simulink model "Aerodynamicsyuan"  (R2017b)
settings: Solver=VariableStepAuto  StartTime=0.0  StopTime=10.0  RelTol=1e-3
values from neighbouring files (symbols this model uses):
  CDAlpha = 0.10031    [aerodata.m]
  CDBeta = 8.0356e-06    [aerodata.m]
  CDDa = 1.3547e-05    [aerodata.m]
  CDDe = 0.020779    [aerodata.m]
  CDDf = 0.031301    [aerodata.m]
  CDDr = 1.437e-05    [aerodata.m]
  CLAlpha = 6.0094    [aerodata.m]
  ClAlpha = -4.2668e-14    [aerodata.m]
  CLBeta = -1.0202e-06    [aerodata.m]
  ClBeta = 0.055654    [aerodata.m]
  CLDa = 2.6815e-06    [aerodata.m]
  ClDa = 0.29533    [aerodata.m]
  CLDe = 0.8867    [aerodata.m]
  CLDf = 2.0336    [aerodata.m]
  CLDr = -3.5351e-06    [aerodata.m]
  ClDr = 0.29533    [aerodata.m]
  CmAlpha = -4.0835    [aerodata.m]
  CmBeta = 5.2248e-06    [aerodata.m]
  CmDa = 1.0717e-06    [aerodata.m]
  CmDe = -2.7271    [aerodata.m]
  CmDf = -0.35441    [aerodata.m]
  CmDr = 1.0717e-06    [aerodata.m]
  CnAlpha = 4.5786e-14    [aerodata.m]
  CnBeta = -0.071639    [aerodata.m]
  CnDa = 0.0089298    [aerodata.m]
  CnDr = -0.10037    [aerodata.m]
  CYAlpha = 8.85452e-14    [aerodata.m]
  CYBeta = -0.25081    [aerodata.m]
  CYDa = 0.0029468    [aerodata.m]
  CYDe = 9.0523e-14    [aerodata.m]
  CYDf = 9.8247e-14    [aerodata.m]
  CYDr = -0.33334    [aerodata.m]
libraries: aerolibatmos2 x1
settings Model: Creator=zht  LastModifiedBy=p'c

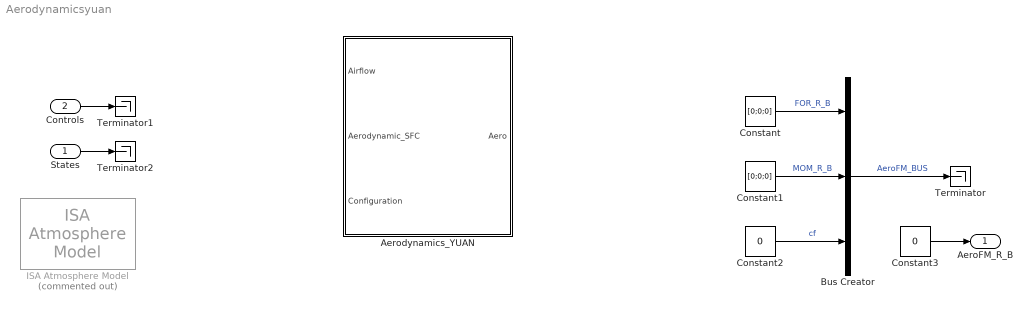
== system Aerodynamicsyuan ==
  States : Inport
  Controls : Inport  Port=2
  Aerodynamics_YUAN : Subsystem
  Bus Creator : BusCreator  Inputs=3
  Constant : Constant  Value=[0;0;0]
  Constant1 : Constant  Value=[0;0;0]
  Constant2 : Constant  Value=0
  Constant3 : Constant  Value=0
  ISA Atmosphere Model : aerolibatmos2/ISA Atmosphere Model  Commented=on  custom=off  g=9.80665  gamma=1.4  R=287.0531  L=0.0065  h_trop=11000  h_strat=20000  rho0=1.225  P0=101325  T0=288.15  h0=0
      settings: SourceProductName=Aerospace Blockset
  Terminator : Terminator
  Terminator1 : Terminator
  Terminator2 : Terminator
  AeroFM_R_B : Outport
  wires:
  Bus Creator/1 -> Terminator/1  "AeroFM_BUS"
  Constant2/1 -> Bus Creator/3  "cf"
  Constant1/1 -> Bus Creator/2  "MOM_R_B"
  Constant/1 -> Bus Creator/1  "FOR_R_B"
  Constant3/1 -> AeroFM_R_B/1
  Controls/1 -> Terminator1/1
  States/1 -> Terminator2/1

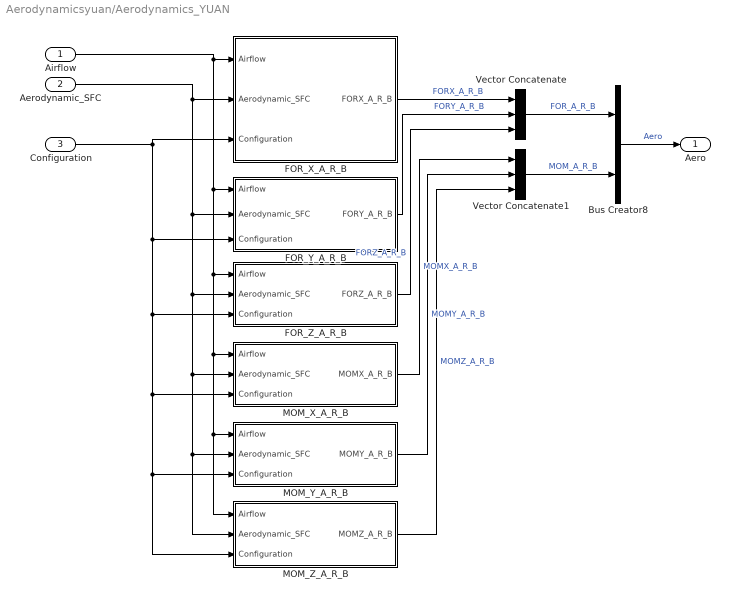
== system Aerodynamicsyuan/Aerodynamics_YUAN ==
  Airflow : Inport  OutDataTypeStr=Bus: Airflow_BUS  BusOutputAsStruct=on
  Aerodynamic_SFC : Inport  Port=2  OutDataTypeStr=Bus: DEF_Aero_SFC_Deflections_BUS  BusOutputAsStruct=on
  Configuration : Inport  Port=3  OutDataTypeStr=Bus: Configuration_BUS  BusOutputAsStruct=on
  Bus Creator8 : BusCreator  Inputs='FOR_A_R_B','MOM_A_R_B'  OutDataTypeStr=Bus: Aero_BUS  NonVirtualBus=on
  FOR_X_A_R_B : Subsystem
  FOR_Y_A_R_B : Subsystem
  FOR_Z_A_R_B : Subsystem
  MOM_X_A_R_B : Subsystem
  MOM_Y_A_R_B : Subsystem
  MOM_Z_A_R_B : Subsystem
  Vector Concatenate : Concatenate  NumInputs=3  Mode=Multidimensional array
  Vector Concatenate1 : Concatenate  NumInputs=3  Mode=Multidimensional array
  Aero : Outport  OutDataTypeStr=Bus: Aero_BUS  BusOutputAsStruct=on
  wires:
  FOR_Y_A_R_B/1(FORY_A_R_B) -> Vector Concatenate/2  "FORY_A_R_B"
  MOM_Z_A_R_B/1(MOMZ_A_R_B) -> Vector Concatenate1/3  "MOMZ_A_R_B"
  MOM_Y_A_R_B/1(MOMY_A_R_B) -> Vector Concatenate1/2  "MOMY_A_R_B"
  Aerodynamic_SFC/1 -> FOR_X_A_R_B/2(Aerodynamic_SFC), FOR_Y_A_R_B/2(Aerodynamic_SFC), FOR_Z_A_R_B/2(Aerodynamic_SFC), MOM_X_A_R_B/2(Aerodynamic_SFC), MOM_Y_A_R_B/2(Aerodynamic_SFC), MOM_Z_A_R_B/2(Aerodynamic_SFC)
  FOR_Z_A_R_B/1(FORZ_A_R_B) -> Vector Concatenate/3  "FORZ_A_R_B"
  Vector Concatenate1/1 -> Bus Creator8/2  "MOM_A_R_B"
  Vector Concatenate/1 -> Bus Creator8/1  "FOR_A_R_B"
  Bus Creator8/1 -> Aero/1  "Aero"
  MOM_X_A_R_B/1(MOMX_A_R_B) -> Vector Concatenate1/1  "MOMX_A_R_B"
  FOR_X_A_R_B/1(FORX_A_R_B) -> Vector Concatenate/1  "FORX_A_R_B"
  Airflow/1 -> FOR_X_A_R_B/1(Airflow), FOR_Y_A_R_B/1(Airflow), FOR_Z_A_R_B/1(Airflow), MOM_X_A_R_B/1(Airflow), MOM_Y_A_R_B/1(Airflow), MOM_Z_A_R_B/1(Airflow)
  Configuration/1 -> FOR_X_A_R_B/3(Configuration), FOR_Y_A_R_B/3(Configuration), FOR_Z_A_R_B/3(Configuration), MOM_X_A_R_B/3(Configuration), MOM_Y_A_R_B/3(Configuration), MOM_Z_A_R_B/3(Configuration)

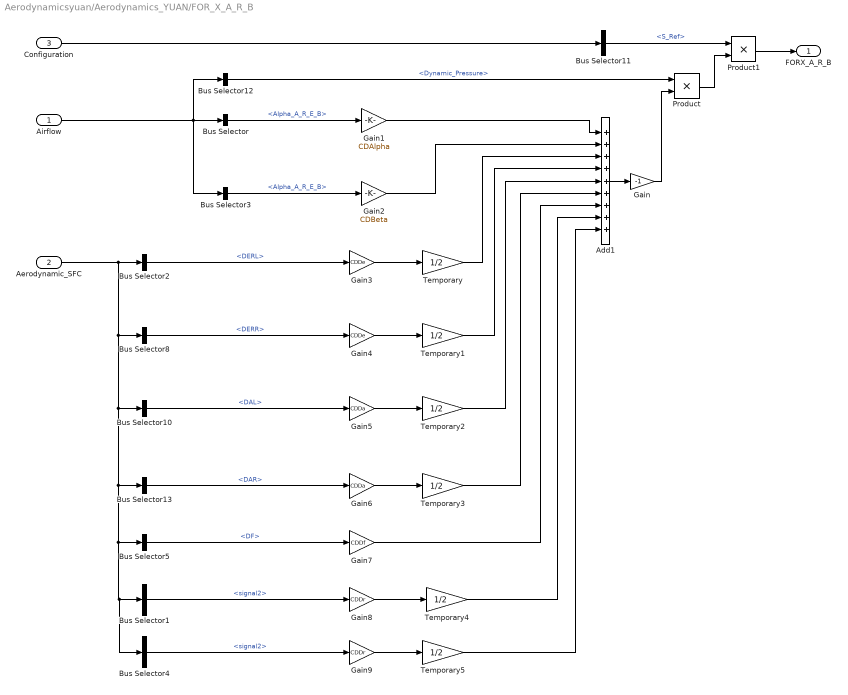
== system Aerodynamicsyuan/Aerodynamics_YUAN/FOR_X_A_R_B ==
  Airflow : Inport  OutDataTypeStr=Bus: Airflow_BUS  BusOutputAsStruct=on
  Aerodynamic_SFC : Inport  Port=2  OutDataTypeStr=Bus: DEF_Aero_SFC_Deflections_BUS  BusOutputAsStruct=on
  Configuration : Inport  Port=3  OutDataTypeStr=Bus: Configuration_BUS  BusOutputAsStruct=on
  Add1 : Sum  Inputs=+++++++++
  Bus Selector : BusSelector  OutputSignals=Alpha_A_R_E_B
  Bus Selector1 : BusSelector  OutputSignals=signal2
  Bus Selector10 : BusSelector  OutputSignals=DAL
  Bus Selector11 : BusSelector  OutputSignals=S_Ref
  Bus Selector12 : BusSelector  OutputSignals=Dynamic_Pressure
  Bus Selector13 : BusSelector  OutputSignals=DAR
  Bus Selector2 : BusSelector  OutputSignals=DERL
  Bus Selector3 : BusSelector  OutputSignals=Alpha_A_R_E_B
  Bus Selector4 : BusSelector  OutputSignals=signal2
  Bus Selector5 : BusSelector  OutputSignals=DF
  Bus Selector8 : BusSelector  OutputSignals=DERR
  Gain : Gain  Gain=-1
  Gain1 : Gain  Gain=CDAlpha
  Gain2 : Gain  Gain=CDBeta
  Gain3 : Gain  Gain=CDDe
  Gain4 : Gain  Gain=CDDe
  Gain5 : Gain  Gain=CDDa
  Gain6 : Gain  Gain=CDDa
  Gain7 : Gain  Gain=CDDf
  Gain8 : Gain  Gain=CDDr
  Gain9 : Gain  Gain=CDDr
  Product : Product
  Product1 : Product
  Temporary{,1..5} (6 alike) : Gain  Gain=1/2
  FORX_A_R_B : Outport  Unit=N  PortDimensions=1
  wires:
  Gain7/1 -> Add1/7
  Gain5/1 -> Temporary2/1
  Gain4/1 -> Temporary1/1
  Bus Selector2/1 -> Gain3/1  "<DERL>"
  Bus Selector8/1 -> Gain4/1  "<DERR>"
  Gain3/1 -> Temporary/1
  Bus Selector10/1 -> Gain5/1  "<DAL>"
  Configuration/1 -> Bus Selector11/1
  Bus Selector12/1 -> Product/1  "<Dynamic_Pressure>"
  Gain2/1 -> Add1/2
  Product1/1 -> FORX_A_R_B/1
  Aerodynamic_SFC/1 -> Bus Selector4/1, Bus Selector1/1, Bus Selector5/1, Bus Selector13/1, Bus Selector10/1, Bus Selector8/1, Bus Selector2/1
  Gain1/1 -> Add1/1
  Temporary1/1 -> Add1/4
  Temporary/1 -> Add1/3
  Gain/1 -> Product/2
  Bus Selector13/1 -> Gain6/1  "<DAR>"
  Bus Selector11/1 -> Product1/1  "<S_Ref>"
  Temporary2/1 -> Add1/5
  Airflow/1 -> Bus Selector12/1, Bus Selector/1, Bus Selector3/1
  Temporary3/1 -> Add1/6
  Gain6/1 -> Temporary3/1
  Bus Selector5/1 -> Gain7/1  "<DF>"
  Bus Selector/1 -> Gain1/1  "<Alpha_A_R_E_B>"
  Add1/1 -> Gain/1
  Bus Selector3/1 -> Gain2/1  "<Alpha_A_R_E_B>"
  Product/1 -> Product1/2
  Bus Selector1/1 -> Gain8/1  "<signal2>"
  Bus Selector4/1 -> Gain9/1  "<signal2>"
  Gain8/1 -> Temporary4/1
  Gain9/1 -> Temporary5/1
  Temporary4/1 -> Add1/8
  Temporary5/1 -> Add1/9

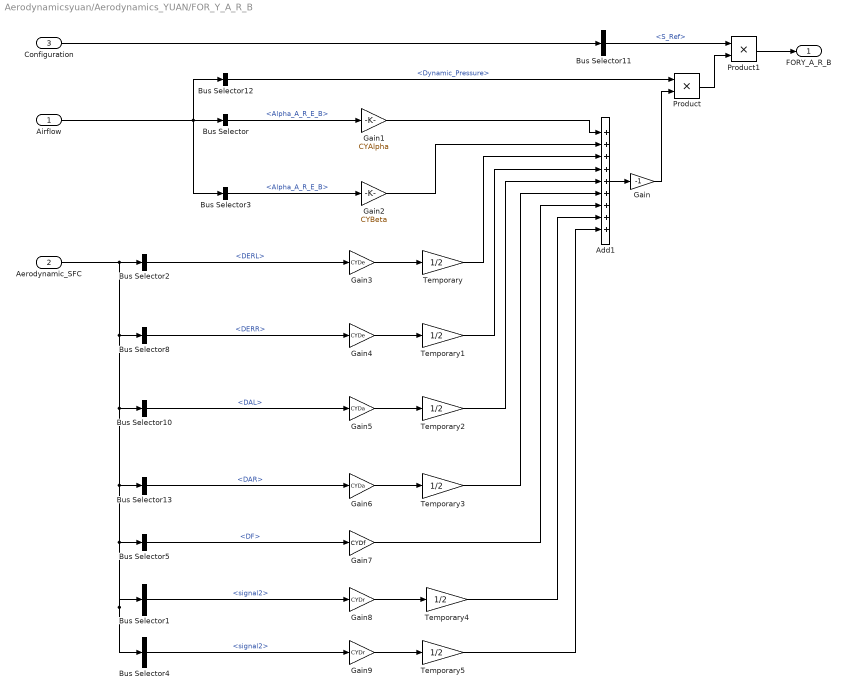
== system Aerodynamicsyuan/Aerodynamics_YUAN/FOR_Y_A_R_B ==
  Airflow : Inport  OutDataTypeStr=Bus: Airflow_BUS  BusOutputAsStruct=on
  Aerodynamic_SFC : Inport  Port=2  OutDataTypeStr=Bus: DEF_Aero_SFC_Deflections_BUS  BusOutputAsStruct=on
  Configuration : Inport  Port=3  OutDataTypeStr=Bus: Configuration_BUS  BusOutputAsStruct=on
  Add1 : Sum  Inputs=+++++++++
  Bus Selector : BusSelector  OutputSignals=Alpha_A_R_E_B
  Bus Selector1 : BusSelector  OutputSignals=signal2
  Bus Selector10 : BusSelector  OutputSignals=DAL
  Bus Selector11 : BusSelector  OutputSignals=S_Ref
  Bus Selector12 : BusSelector  OutputSignals=Dynamic_Pressure
  Bus Selector13 : BusSelector  OutputSignals=DAR
  Bus Selector2 : BusSelector  OutputSignals=DERL
  Bus Selector3 : BusSelector  OutputSignals=Alpha_A_R_E_B
  Bus Selector4 : BusSelector  OutputSignals=signal2
  Bus Selector5 : BusSelector  OutputSignals=DF
  Bus Selector8 : BusSelector  OutputSignals=DERR
  Gain : Gain  Gain=-1
  Gain1 : Gain  Gain=CYAlpha
  Gain2 : Gain  Gain=CYBeta
  Gain3 : Gain  Gain=CYDe
  Gain4 : Gain  Gain=CYDe
  Gain5 : Gain  Gain=CYDa
  Gain6 : Gain  Gain=CYDa
  Gain7 : Gain  Gain=CYDf
  Gain8 : Gain  Gain=CYDr
  Gain9 : Gain  Gain=CYDr
  Product : Product
  Product1 : Product
  Temporary{,1..5} (6 alike) : Gain  Gain=1/2
  FORY_A_R_B : Outport  Unit=N  PortDimensions=1
  wires:
  Gain8/1 -> Temporary4/1
  Bus Selector/1 -> Gain1/1  "<Alpha_A_R_E_B>"
  Bus Selector5/1 -> Gain7/1  "<DF>"
  Bus Selector2/1 -> Gain3/1  "<DERL>"
  Gain7/1 -> Add1/7
  Temporary4/1 -> Add1/8
  Gain2/1 -> Add1/2
  Add1/1 -> Gain/1
  Bus Selector13/1 -> Gain6/1  "<DAR>"
  Temporary3/1 -> Add1/6
  Temporary/1 -> Add1/3
  Temporary1/1 -> Add1/4
  Airflow/1 -> Bus Selector12/1, Bus Selector/1, Bus Selector3/1
  Bus Selector8/1 -> Gain4/1  "<DERR>"
  Gain5/1 -> Temporary2/1
  Product1/1 -> FORY_A_R_B/1
  Bus Selector11/1 -> Product1/1  "<S_Ref>"
  Bus Selector4/1 -> Gain9/1  "<signal2>"
  Gain9/1 -> Temporary5/1
  Gain/1 -> Product/2
  Bus Selector12/1 -> Product/1  "<Dynamic_Pressure>"
  Gain4/1 -> Temporary1/1
  Gain6/1 -> Temporary3/1
  Temporary2/1 -> Add1/5
  Bus Selector1/1 -> Gain8/1  "<signal2>"
  Configuration/1 -> Bus Selector11/1
  Bus Selector10/1 -> Gain5/1  "<DAL>"
  Temporary5/1 -> Add1/9
  Product/1 -> Product1/2
  Gain3/1 -> Temporary/1
  Aerodynamic_SFC/1 -> Bus Selector4/1, Bus Selector1/1, Bus Selector5/1, Bus Selector13/1, Bus Selector10/1, Bus Selector8/1, Bus Selector2/1
  Gain1/1 -> Add1/1
  Bus Selector3/1 -> Gain2/1  "<Alpha_A_R_E_B>"

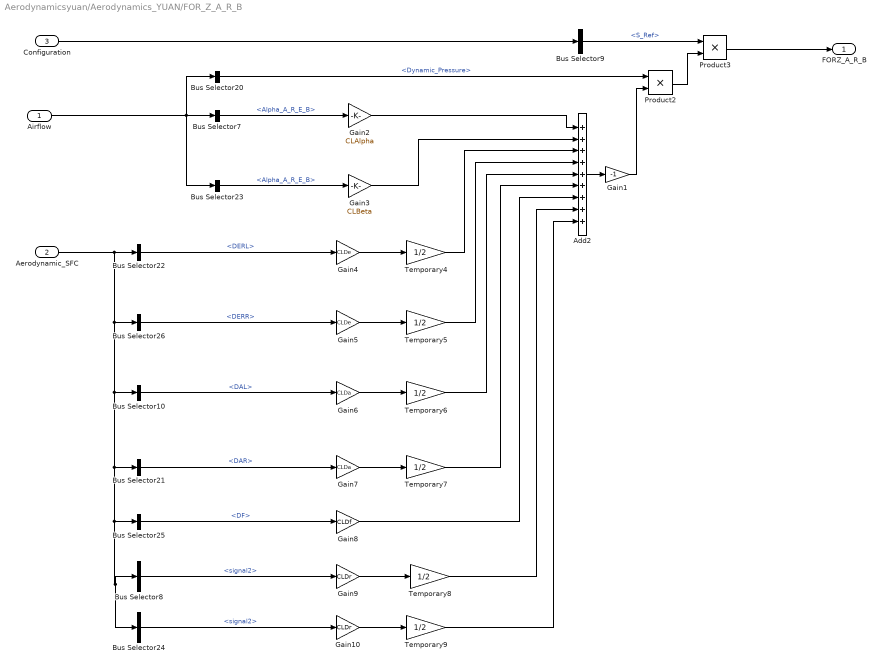
== system Aerodynamicsyuan/Aerodynamics_YUAN/FOR_Z_A_R_B ==
  Airflow : Inport  OutDataTypeStr=Bus: Airflow_BUS  BusOutputAsStruct=on
  Aerodynamic_SFC : Inport  Port=2  OutDataTypeStr=Bus: DEF_Aero_SFC_Deflections_BUS  BusOutputAsStruct=on
  Configuration : Inport  Port=3  OutDataTypeStr=Bus: Configuration_BUS  BusOutputAsStruct=on
  Add2 : Sum  Inputs=+++++++++
  Bus Selector10 : BusSelector  OutputSignals=DAL
  Bus Selector20 : BusSelector  OutputSignals=Dynamic_Pressure
  Bus Selector21 : BusSelector  OutputSignals=DAR
  Bus Selector22 : BusSelector  OutputSignals=DERL
  Bus Selector23 : BusSelector  OutputSignals=Alpha_A_R_E_B
  Bus Selector24 : BusSelector  OutputSignals=signal2
  Bus Selector25 : BusSelector  OutputSignals=DF
  Bus Selector26 : BusSelector  OutputSignals=DERR
  Bus Selector7 : BusSelector  OutputSignals=Alpha_A_R_E_B
  Bus Selector8 : BusSelector  OutputSignals=signal2
  Bus Selector9 : BusSelector  OutputSignals=S_Ref
  Gain1 : Gain  Gain=-1
  Gain10 : Gain  Gain=CLDr
  Gain2 : Gain  Gain=CLAlpha
  Gain3 : Gain  Gain=CLBeta
  Gain4 : Gain  Gain=CLDe
  Gain5 : Gain  Gain=CLDe
  Gain6 : Gain  Gain=CLDa
  Gain7 : Gain  Gain=CLDa
  Gain8 : Gain  Gain=CLDf
  Gain9 : Gain  Gain=CLDr
  Product2 : Product
  Product3 : Product
  Temporary{4..9} (6 alike) : Gain  Gain=1/2
  FORZ_A_R_B : Outport  Unit=N  PortDimensions=1
  wires:
  Gain5/1 -> Temporary5/1
  Aerodynamic_SFC/1 -> Bus Selector24/1, Bus Selector8/1, Bus Selector25/1, Bus Selector21/1, Bus Selector10/1, Bus Selector26/1, Bus Selector22/1
  Bus Selector20/1 -> Product2/1  "<Dynamic_Pressure>"
  Product2/1 -> Product3/2
  Gain1/1 -> Product2/2
  Temporary6/1 -> Add2/5
  Configuration/1 -> Bus Selector9/1
  Temporary9/1 -> Add2/9
  Temporary7/1 -> Add2/6
  Temporary4/1 -> Add2/3
  Bus Selector10/1 -> Gain6/1  "<DAL>"
  Gain7/1 -> Temporary7/1
  Bus Selector21/1 -> Gain7/1  "<DAR>"
  Add2/1 -> Gain1/1
  Gain4/1 -> Temporary4/1
  Gain3/1 -> Add2/2
  Temporary8/1 -> Add2/8
  Gain8/1 -> Add2/7
  Bus Selector22/1 -> Gain4/1  "<DERL>"
  Bus Selector25/1 -> Gain8/1  "<DF>"
  Bus Selector7/1 -> Gain2/1  "<Alpha_A_R_E_B>"
  Gain9/1 -> Temporary8/1
  Gain10/1 -> Temporary9/1
  Bus Selector8/1 -> Gain9/1  "<signal2>"
  Gain2/1 -> Add2/1
  Bus Selector24/1 -> Gain10/1  "<signal2>"
  Bus Selector9/1 -> Product3/1  "<S_Ref>"
  Gain6/1 -> Temporary6/1
  Bus Selector26/1 -> Gain5/1  "<DERR>"
  Bus Selector23/1 -> Gain3/1  "<Alpha_A_R_E_B>"
  Product3/1 -> FORZ_A_R_B/1
  Temporary5/1 -> Add2/4
  Airflow/1 -> Bus Selector20/1, Bus Selector7/1, Bus Selector23/1

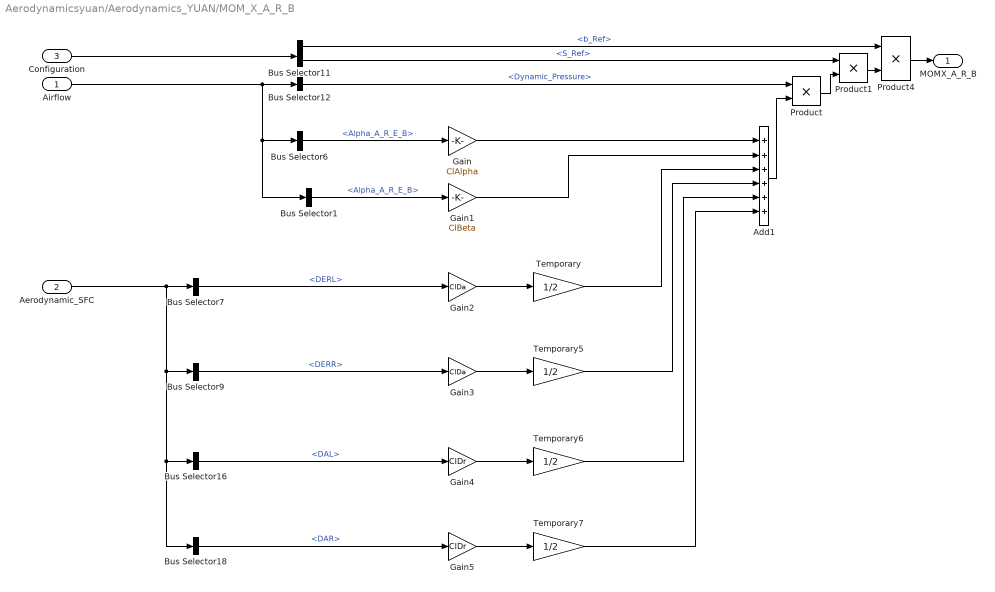
== system Aerodynamicsyuan/Aerodynamics_YUAN/MOM_X_A_R_B ==
  Airflow : Inport  OutDataTypeStr=Bus: Airflow_BUS  BusOutputAsStruct=on
  Aerodynamic_SFC : Inport  Port=2  OutDataTypeStr=Bus: DEF_Aero_SFC_Deflections_BUS  BusOutputAsStruct=on
  Configuration : Inport  Port=3  OutDataTypeStr=Bus: Configuration_BUS  BusOutputAsStruct=on
  Add1 : Sum  Inputs=++++++
  Bus Selector1 : BusSelector  OutputSignals=Alpha_A_R_E_B
  Bus Selector11 : BusSelector  OutputSignals=b_Ref,S_Ref
  Bus Selector12 : BusSelector  OutputSignals=Dynamic_Pressure
  Bus Selector16 : BusSelector  OutputSignals=DAL
  Bus Selector18 : BusSelector  OutputSignals=DAR
  Bus Selector6 : BusSelector  OutputSignals=Alpha_A_R_E_B
  Bus Selector7 : BusSelector  OutputSignals=DERL
  Bus Selector9 : BusSelector  OutputSignals=DERR
  Gain : Gain  Gain=ClAlpha
  Gain1 : Gain  Gain=ClBeta
  Gain2 : Gain  Gain=ClDa
  Gain3 : Gain  Gain=ClDa
  Gain4 : Gain  Gain=ClDr
  Gain5 : Gain  Gain=ClDr
  Product : Product
  Product1 : Product
  Product4 : Product
  Temporary{,5..7} (4 alike) : Gain  Gain=1/2
  MOMX_A_R_B : Outport  Unit=N*m  PortDimensions=1
  wires:
  Add1/1 -> Product/2
  Bus Selector12/1 -> Product/1  "<Dynamic_Pressure>"
  Product/1 -> Product1/2
  Bus Selector11/2 -> Product1/1  "<S_Ref>"
  Bus Selector11/1 -> Product4/1  "<b_Ref>"
  Product1/1 -> Product4/2
  Product4/1 -> MOMX_A_R_B/1
  Configuration/1 -> Bus Selector11/1
  Bus Selector6/1 -> Gain/1  "<Alpha_A_R_E_B>"
  Gain2/1 -> Temporary/1
  Bus Selector7/1 -> Gain2/1  "<DERL>"
  Bus Selector9/1 -> Gain3/1  "<DERR>"
  Gain3/1 -> Temporary5/1
  Bus Selector16/1 -> Gain4/1  "<DAL>"
  Gain4/1 -> Temporary6/1
  Gain5/1 -> Temporary7/1
  Bus Selector18/1 -> Gain5/1  "<DAR>"
  Airflow/1 -> Bus Selector1/1, Bus Selector6/1, Bus Selector12/1
  Aerodynamic_SFC/1 -> Bus Selector9/1, Bus Selector16/1, Bus Selector18/1, Bus Selector7/1
  Gain/1 -> Add1/1
  Gain1/1 -> Add1/2
  Temporary/1 -> Add1/3
  Temporary5/1 -> Add1/4
  Temporary6/1 -> Add1/5
  Temporary7/1 -> Add1/6
  Bus Selector1/1 -> Gain1/1  "<Alpha_A_R_E_B>"

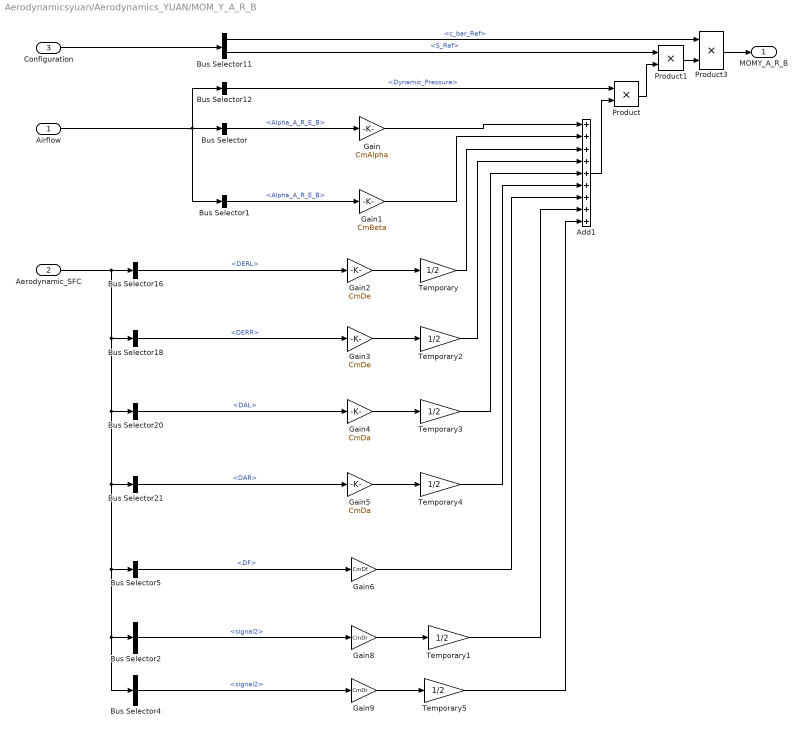
== system Aerodynamicsyuan/Aerodynamics_YUAN/MOM_Y_A_R_B ==
  Airflow : Inport  OutDataTypeStr=Bus: Airflow_BUS  BusOutputAsStruct=on
  Aerodynamic_SFC : Inport  Port=2  OutDataTypeStr=Bus: DEF_Aero_SFC_Deflections_BUS  BusOutputAsStruct=on
  Configuration : Inport  Port=3  OutDataTypeStr=Bus: Configuration_BUS  BusOutputAsStruct=on
  Add1 : Sum  Inputs=+++++++++
  Bus Selector : BusSelector  OutputSignals=Alpha_A_R_E_B
  Bus Selector1 : BusSelector  OutputSignals=Alpha_A_R_E_B
  Bus Selector11 : BusSelector  OutputSignals=c_bar_Ref,S_Ref
  Bus Selector12 : BusSelector  OutputSignals=Dynamic_Pressure
  Bus Selector16 : BusSelector  OutputSignals=DERL
  Bus Selector18 : BusSelector  OutputSignals=DERR
  Bus Selector2 : BusSelector  OutputSignals=signal2
  Bus Selector20 : BusSelector  OutputSignals=DAL
  Bus Selector21 : BusSelector  OutputSignals=DAR
  Bus Selector4 : BusSelector  OutputSignals=signal2
  Bus Selector5 : BusSelector  OutputSignals=DF
  Gain : Gain  Gain=CmAlpha
  Gain1 : Gain  Gain=CmBeta
  Gain2 : Gain  Gain=CmDe
  Gain3 : Gain  Gain=CmDe
  Gain4 : Gain  Gain=CmDa
  Gain5 : Gain  Gain=CmDa
  Gain6 : Gain  Gain=CmDf
  Gain8 : Gain  Gain=CmDr
  Gain9 : Gain  Gain=CmDr
  Product : Product
  Product1 : Product
  Product3 : Product
  Temporary{,1..5} (6 alike) : Gain  Gain=1/2
  MOMY_A_R_B : Outport  Unit=N*m  PortDimensions=1
  wires:
  Bus Selector/1 -> Gain/1  "<Alpha_A_R_E_B>"
  Bus Selector5/1 -> Gain6/1  "<DF>"
  Add1/1 -> Product/2
  Bus Selector12/1 -> Product/1  "<Dynamic_Pressure>"
  Product/1 -> Product1/2
  Bus Selector11/2 -> Product1/1  "<S_Ref>"
  Product1/1 -> Product3/2
  Configuration/1 -> Bus Selector11/1
  Bus Selector11/1 -> Product3/1  "<c_bar_Ref>"
  Product3/1 -> MOMY_A_R_B/1
  Gain2/1 -> Temporary/1
  Bus Selector16/1 -> Gain2/1  "<DERL>"
  Bus Selector18/1 -> Gain3/1  "<DERR>"
  Gain3/1 -> Temporary2/1
  Gain4/1 -> Temporary3/1
  Bus Selector20/1 -> Gain4/1  "<DAL>"
  Airflow/1 -> Bus Selector12/1, Bus Selector/1, Bus Selector1/1
  Bus Selector21/1 -> Gain5/1  "<DAR>"
  Gain5/1 -> Temporary4/1
  Gain/1 -> Add1/1
  Gain1/1 -> Add1/2
  Temporary/1 -> Add1/3
  Temporary2/1 -> Add1/4
  Temporary3/1 -> Add1/5
  Temporary4/1 -> Add1/6
  Gain6/1 -> Add1/7
  Bus Selector1/1 -> Gain1/1  "<Alpha_A_R_E_B>"
  Gain9/1 -> Temporary5/1
  Gain8/1 -> Temporary1/1
  Bus Selector4/1 -> Gain9/1  "<signal2>"
  Aerodynamic_SFC/1 -> Bus Selector5/1, Bus Selector4/1, Bus Selector2/1, Bus Selector21/1, Bus Selector20/1, Bus Selector18/1, Bus Selector16/1
  Bus Selector2/1 -> Gain8/1  "<signal2>"
  Temporary1/1 -> Add1/8
  Temporary5/1 -> Add1/9

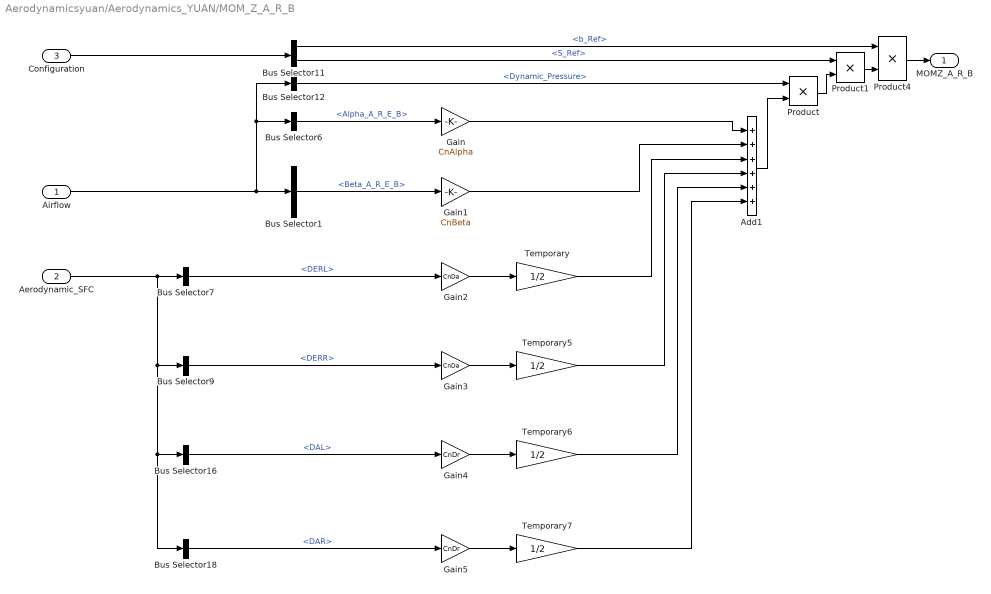
== system Aerodynamicsyuan/Aerodynamics_YUAN/MOM_Z_A_R_B ==
  Airflow : Inport  OutDataTypeStr=Bus: Airflow_BUS  BusOutputAsStruct=on
  Aerodynamic_SFC : Inport  Port=2  OutDataTypeStr=Bus: DEF_Aero_SFC_Deflections_BUS  BusOutputAsStruct=on
  Configuration : Inport  Port=3  OutDataTypeStr=Bus: Configuration_BUS  BusOutputAsStruct=on
  Add1 : Sum  Inputs=++++++
  Bus Selector1 : BusSelector  OutputSignals=Beta_A_R_E_B
  Bus Selector11 : BusSelector  OutputSignals=b_Ref,S_Ref
  Bus Selector12 : BusSelector  OutputSignals=Dynamic_Pressure
  Bus Selector16 : BusSelector  OutputSignals=DAL
  Bus Selector18 : BusSelector  OutputSignals=DAR
  Bus Selector6 : BusSelector  OutputSignals=Alpha_A_R_E_B
  Bus Selector7 : BusSelector  OutputSignals=DERL
  Bus Selector9 : BusSelector  OutputSignals=DERR
  Gain : Gain  Gain=CnAlpha
  Gain1 : Gain  Gain=CnBeta
  Gain2 : Gain  Gain=CnDa
  Gain3 : Gain  Gain=CnDa
  Gain4 : Gain  Gain=CnDr
  Gain5 : Gain  Gain=CnDr
  Product : Product
  Product1 : Product
  Product4 : Product
  Temporary{,5..7} (4 alike) : Gain  Gain=1/2
  MOMZ_A_R_B : Outport  Unit=N*m  PortDimensions=1
  wires:
  Bus Selector11/2 -> Product1/1  "<S_Ref>"
  Bus Selector1/1 -> Gain1/1  "<Beta_A_R_E_B>"
  Add1/1 -> Product/2
  Product/1 -> Product1/2
  Product1/1 -> Product4/2
  Bus Selector11/1 -> Product4/1  "<b_Ref>"
  Product4/1 -> MOMZ_A_R_B/1
  Bus Selector12/1 -> Product/1  "<Dynamic_Pressure>"
  Bus Selector6/1 -> Gain/1  "<Alpha_A_R_E_B>"
  Bus Selector7/1 -> Gain2/1  "<DERL>"
  Gain2/1 -> Temporary/1
  Gain3/1 -> Temporary5/1
  Bus Selector9/1 -> Gain3/1  "<DERR>"
  Bus Selector16/1 -> Gain4/1  "<DAL>"
  Gain4/1 -> Temporary6/1
  Gain5/1 -> Temporary7/1
  Bus Selector18/1 -> Gain5/1  "<DAR>"
  Airflow/1 -> Bus Selector1/1, Bus Selector6/1, Bus Selector12/1
  Aerodynamic_SFC/1 -> Bus Selector7/1, Bus Selector9/1, Bus Selector16/1, Bus Selector18/1
  Gain/1 -> Add1/1
  Gain1/1 -> Add1/2
  Temporary/1 -> Add1/3
  Temporary5/1 -> Add1/4
  Temporary6/1 -> Add1/5
  Temporary7/1 -> Add1/6
  Configuration/1 -> Bus Selector11/1
